simulink model "modelReferenceTest_MR"  (Simulink 7.6)
settings: Solver=FixedStepDiscrete  StartTime=0.0  StopTime=10.0  FixedStep=1  RelTol=1e-3
settings Model: Creator=c2wt  LastModifiedBy=c2wt
settings OptimizationCC: InlineParams=on

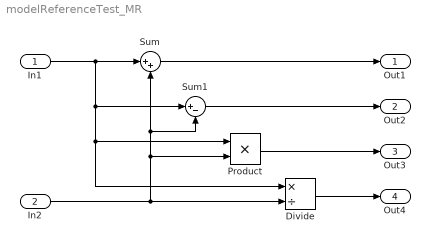
== system modelReferenceTest_MR ==
  In1 : Inport
  In2 : Inport  Port=2
  Divide : Product  Inputs=*/
  Product : Product  RndMeth=Zero
  Sum : Sum  Inputs=|++
  Sum1 : Sum  Inputs=|+-
  Out1 : Outport
  Out2 : Outport  Port=2
  Out3 : Outport  Port=3
  Out4 : Outport  Port=4
  wires:
  In1/1 -> Sum/1, Sum1/1, Product/1, Divide/1
  In2/1 -> Sum/2, Sum1/2, Product/2, Divide/2
  Sum/1 -> Out1/1
  Sum1/1 -> Out2/1
  Product/1 -> Out3/1
  Divide/1 -> Out4/1
